simulink model "servomoteur"  (R2020a)
settings: Solver=FixedStepDiscrete  StartTime=0.00  StopTime=10.0  FixedStep=0.01  RelTol=1e-3  EnableMultiTasking=on
libraries: arduinolib x2
settings Model: SILPILModeSetting=veronly  ExtModeTrigDuration=2  Creator=pc  LastModifiedBy=pc
settings OptimizationCC: EnhancedBackFolding=on  PassReuseOutputArgsAs=Individual arguments  ZeroExternalMemoryAtStartup=off  ZeroInternalMemoryAtStartup=off  MaxStackSize=64  OptimizeBlockOrder=speed  DifferentSizesBufferReuse=on  OptimizationCustomize=off  EfficientTunableParamExpr=on
settings DebuggingCC: ParameterTunabilityLossMsg=error
settings HardwareCC: ProdBitPerInt=16  ProdBitPerPointer=16  ProdBitPerSizeT=16  ProdBitPerPtrDiffT=16  ProdLargestAtomicFloat=None  ProdWordSize=8  ProdHWDeviceType=Atmel->AVR
settings SFSimCC: MATLABDynamicMemAlloc=off
settings RTWCC: SystemTargetFile=ert.tlc  HardwareBoard=Arduino Uno  TLCOptions=-aInlineSetEventsForThisBaseRateFcn=TLC_FALSE -aSuppressMultiTaskScheduler=TLC_FALSE -aRateBasedStepFcn=1  TemplateMakefile=ert_default_tmf  Toolchain=Arduino AVR  BuildConfiguration=Faster Runs
settings CodeAppCC: ForceParamTrailComments=on  IgnoreCustomStorageClasses=off  OperatorAnnotations=on  SimulinkDataObjDesc=on  SFDataObjDesc=on  InsertBlockDesc=on
settings ERTTargetCC: SupportContinuousTime=on  SupportVariableSizeSignals=on  ExtModeStaticAllocSize=250

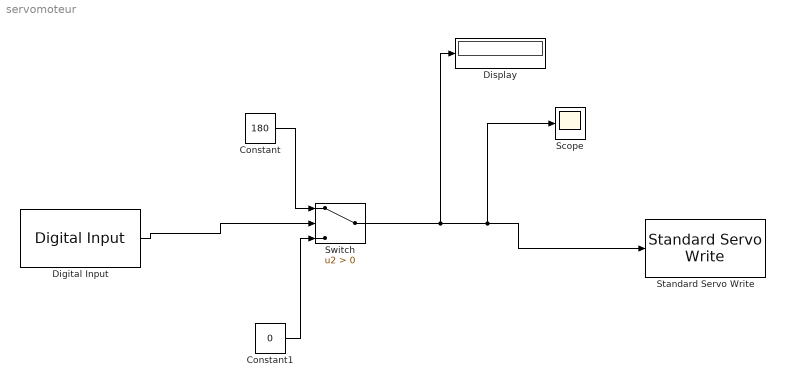
== system servomoteur ==
  Constant : Constant  Value=180
  Constant1 : Constant  Value=0
  Digital Input : arduinolib/Digital Input  pinNumber=2  Direction=input  SampleTime=0.1  blockPlatform=arduino
  Display : Display
  Scope : Scope
  Standard Servo Write : arduinolib/Standard Servo Write  pinNumber=4  ServoIndex=0  blockPlatform=ARDUINO
  Switch : Switch  Criteria=u2 > Threshold
  wires:
  Digital Input/1 -> Switch/2
  Switch/1 -> Display/1, Scope/1, Standard Servo Write/1
  Constant1/1 -> Switch/3
  Constant/1 -> Switch/1
